simulink model "Practica_3"  (R2020b)
settings: Solver=VariableStepAuto  StartTime=0.0  StopTime=120  RelTol=1e-3
undefined symbols (not defined in the file or in its folder): serial
libraries: instrumentlib x2
settings Model: Creator=Dell  LastModifiedBy=Dell

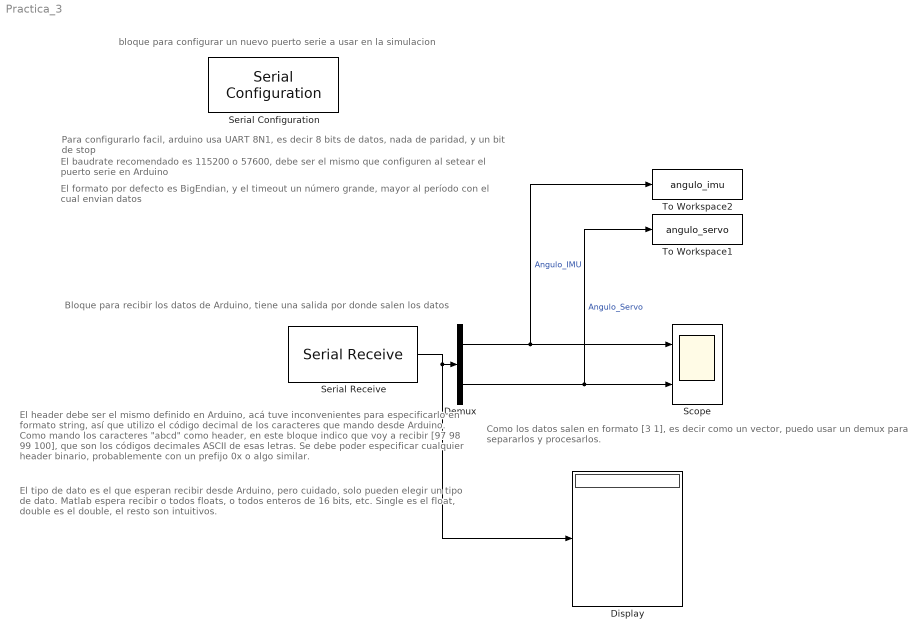
== system Practica_3 ==
  note: Como los datos salen en formato [3 1], es decir como un vector, puedo usar un demux para separarlos y procesarlos.
  note: El header debe ser el mismo definido en Arduino, acá tuve inconvenientes para especificarlo en formato string, así que utilizo el código decimal de los caracteres que mando desde Arduino. Como mando los caracteres "abcd" como header, en este bloque indico que voy a recibir [97 98 99 100], que son los códigos decimales ASCII de esas letras. Se debe poder especificar cualquier header binario, probablemente con un prefijo 0x o algo similar.
  note: El formato por defecto es BigEndian, y el timeout un número grande, mayor al período con el cual envian datos
  note: Bloque para recibir los datos de Arduino, tiene una salida por donde salen los datos
  note: El tipo de dato es el que esperan recibir desde Arduino, pero cuidado, solo pueden elegir un tipo de dato. Matlab espera recibir o todos floats, o todos enteros de 16 bits, etc. Single es el float, double es el double, el resto son intuitivos.
  note: bloque para configurar un nuevo puerto serie a usar en la simulacion
  note: El baudrate recomendado es 115200 o 57600, debe ser el mismo que configuren al setear el puerto serie en Arduino
  note: Para configurarlo facil, arduino usa UART 8N1, es decir 8 bits de datos, nada de paridad, y un bit de stop
  Demux : Demux  Outputs=2
  Display : Display
  Scope : Scope  NumInputPorts=2
  Serial Configuration : instrumentlib/Serial Configuration  Priority=-200000  ComPortMenu=<Please select a port...>  ComPort=COM9  ObjConstructor=serial('COM9');  BaudRate=115200  DataBits=8  Parity=none  StopBits=1  FlowControl=none  Timeout=10  ByteOrder=LittleEndian
  Serial Receive : instrumentlib/Serial Receive  Priority=1  ComPortMenu=<Please select a port...>  ComPort=COM9  ObjConstructor=serial('COM9');  Header=abcd  Terminator=<none>  DataSize="[2  1]"  DataType=single  EnableBlockingMode=on  ActionDataUnavailable=Output last received value  CustomValue=0  SampleTime=0.02
  To Workspace1 : ToWorkspace  VariableName=angulo_servo  SampleTime=-1
      settings: Save2DSignal=2-D array (concatenate along first dimension)
  To Workspace2 : ToWorkspace  VariableName=angulo_imu  SampleTime=-1
      settings: Save2DSignal=2-D array (concatenate along first dimension)
  wires:
  Serial Receive/1 -> Display/1, Demux/1
  Demux/2 -> To Workspace1/1, Scope/2  "Angulo_Servo"
  Demux/1 -> To Workspace2/1, Scope/1  "Angulo_IMU"
